simulink model "Praktikum03Grupp09"  (R2023b)
settings: Solver=VariableStepAuto  StartTime=0.0  StopTime=Inf  RelTol=1e-3
model workspace (MAT data in the model file):
  M = 16
  Ts = 5e-08
undefined symbols (not defined in the file): doppler
libraries: commchan3 x6, commrflib2 x6, dspsrcs4 x4, dspxfrm3 x3, commrandsrc3 x2, dspsigops x2, commdigbbndam3 x2, dspstat3 x1, dspmathops x1
settings Model: Creator=suttarar@hu-berlin.de  LastModifiedBy=suttarar@hu-berlin.de

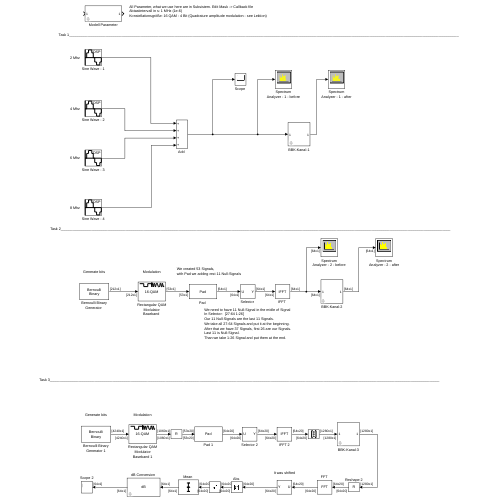
[thumbnail: Simulink's stored preview of the top-level diagram]
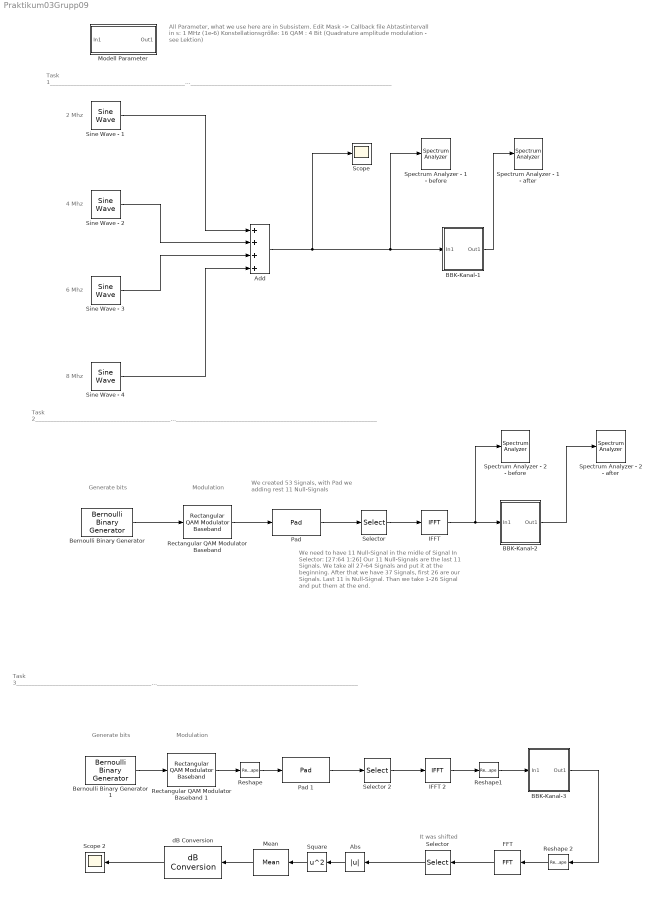
== system Praktikum03Grupp09 ==
  note: It was shifted
  note: Task 1________________________________________________________________________________________________________________________________________________________________________________________________
  note: We need to have 11 Null-Signal in the midle of Signal
      | In Selector:  [27:64 1:26]
      | Our 11 Null-Signals are the last 11 Signals.
      | We take all 27-64 Signals and put it at the beginning.
      | After that we have 37 Signals, first 26 are our Signals.
      | Last 11 is Null-Signal.
      | Than we take 1-26 Signal and put them at the end.
  note: We created 53 Signals,
      | with Pad we adding rest 11 Null-Signals
  note: 2 Mhz
  note: 4 Mhz
  note: 6 Mhz
  note: 8 Mhz
  note: All Parameter, what we use here are in Subsistem. Edit Mask -> Callback file
      | Abtastintervall in s: 1 MHz (1e-6)
      | Konstellationsgröße: 16 QAM : 4 Bit (Quadrature amplitude modulation - see Lektion)
  note: Modulation
  note: Generate bits
  note: Task 2________________________________________________________________________________________________________________________________________________________________________________________________
  note: Generate bits
  note: Task 3________________________________________________________________________________________________________________________________________________________________________________________________
  note: Modulation
  "Abs " : Abs  SaturateOnIntegerOverflow=off
  "Add " : Sum  Inputs=++++
  BBK-Kanal-1 : Subsystem  mask{MaxDoppler=10, PathDelays=[0 100]*1e-9, PathGains=[0 -3], EnableMultipath=1, PathLoss=0, FrequencyOffset=0, PhaseOffset=0, SNR=20}
      mask prompts: MaxDoppler "Dopplerverschiebung"; PathDelays "Pfadverzoergerungen"; PathGains "Pfadverstaerkungen"; EnableMultipath "SwitchBlock"; PathLoss "Pfadverlust"; FrequencyOffset "Frequenzverschiebung"; PhaseOffset "Phasenverschiebung"; SNR "AWG-Rauschen"
  BBK-Kanal-2 : Subsystem  mask{MaxDoppler=10, PathDelays=[0 100]*1e-9, PathGains=[0 -3], EnableMultipath=1, PathLoss=0, FrequencyOffset=0, PhaseOffset=0, SNR=20}
      mask prompts: MaxDoppler "Dopplerverschiebung"; PathDelays "Pfadverzoergerungen"; PathGains "Pfadverstaerkungen"; EnableMultipath "SwitchBlock"; PathLoss "Pfadverlust"; FrequencyOffset "Frequenzverschiebung"; PhaseOffset "Phasenverschiebung"; SNR "AWG-Rauschen"
  BBK-Kanal-3 : Subsystem  mask{MaxDoppler=10, PathDelays=[0 100]*1e-9, PathGains=[0 -3], EnableMultipath=1, PathLoss=0, FrequencyOffset=0, PhaseOffset=0, SNR=20}
      mask prompts: MaxDoppler "Dopplerverschiebung"; PathDelays "Pfadverzoergerungen"; PathGains "Pfadverstaerkungen"; EnableMultipath "SwitchBlock"; PathLoss "Pfadverlust"; FrequencyOffset "Frequenzverschiebung"; PhaseOffset "Phasenverschiebung"; SNR "AWG-Rauschen"
  "Bernoulli Binary Generator " : commrandsrc3/Bernoulli Binary Generator  ProbabilityOfZero=0.5  SeedSource=Auto  Seed=0  SampleTime=Ts*64/(log2(M)*53)  SamplesPerFrame=log2(M)*53  OutputDataType=double  SimulateUsing=Interpreted execution
  Bernoulli Binary Generator 1 : commrandsrc3/Bernoulli Binary Generator  ProbabilityOfZero=0.5  SeedSource=Auto  Seed=0  SampleTime=Ts*64/(log2(M)*53)  SamplesPerFrame=log2(M)*53 * 20  OutputDataType=double  SimulateUsing=Interpreted execution
  "FFT " : dspxfrm3/FFT  FFTImplementation=Auto  CompMethod=Table lookup  TableOpt=NEW  TableOptActive=Speed  BitRevOrder=off  Normalize=off  InheritFFTLength=on  FFTLength=64  WrapInput=on  roundingMode=Floor  overflowMode=off  firstCoeffDataTypeStr=Inherit: Same word length as input  firstCoeffLastDataTypeStr=Inherit: Same word length as input  outputMin=[]  outputMax=[]
  "IFFT " : dspxfrm3/IFFT  FFTImplementation=Auto  CompMethod=Table lookup  TableOpt=NEW  TableOptActive=Speed  BitRevOrder=off  cs_in=off  Normalize=on  InheritFFTLength=on  FFTLength=64  WrapInput=on  mode=Complex  outSamplingMode=Sample based  roundingMode=Floor  overflowMode=off  firstCoeffDataTypeStr=Inherit: Same word length as input  firstCoeffLastDataTypeStr=Inherit: Same word length as input  outputMin=[]  outputMax=[]
  IFFT 2 : dspxfrm3/IFFT  FFTImplementation=Auto  CompMethod=Table lookup  TableOpt=NEW  TableOptActive=Speed  BitRevOrder=off  cs_in=off  Normalize=on  InheritFFTLength=on  FFTLength=64  WrapInput=on  mode=Complex  outSamplingMode=Sample based  roundingMode=Floor  overflowMode=off  firstCoeffDataTypeStr=Inherit: Same word length as input  firstCoeffLastDataTypeStr=Inherit: Same word length as input  outputMin=[]  outputMax=[]
  "Mean " : dspstat3/Mean  run=off  InputProcessing=Columns as channels (frame based)  reset_popup=None  directionMode=Each row  dimension=1  roiEnable=off  roiType=Rectangles  roiPortion=Entire ROI  roiOutput=Individual statistics for each ROI  roiFlag=off  roundingMode=Floor  overflowMode=off  outputDataTypeStr=Inherit: Same as accumulator  outputMin=[]  outputMax=[]  outputLastDataTypeStr=Inherit: Same as accumulator
  Modell Parameter : Subsystem  mask{Ts=1/20e6, M=16}
      mask prompts: Ts "Abtastintervall in s"; M "Konstellationsgröße"
  "Pad " : dspsigops/Pad  padAlong=Columns  dimsToPad=1  valSrc=Specify via dialog  padVal=0  spec=Output size  padNumOutRowsSpecMethod=User-specified  numOutRows=64  padNumOutColsSpecMethod=User-specified  numOutCols=1  isVarDimsMode=off  padBeginning=0  padEnd=0  outSizeMode=User-specified  outSize=1  padSigAt=End  trunc_flag=None  roundingMode=Floor  overflowMode=off  truncOrWrapMode=Truncate  wrap_flag=None
  Pad 1 : dspsigops/Pad  padAlong=Columns  dimsToPad=1  valSrc=Specify via dialog  padVal=0  spec=Output size  padNumOutRowsSpecMethod=User-specified  numOutRows=64  padNumOutColsSpecMethod=User-specified  numOutCols=1  isVarDimsMode=off  padBeginning=0  padEnd=0  outSizeMode=User-specified  outSize=1  padSigAt=End  trunc_flag=None  roundingMode=Floor  overflowMode=off  truncOrWrapMode=Truncate  wrap_flag=None
  "Rectangular QAM Modulator Baseband " : commdigbbndam3/Rectangular QAM Modulator Baseband  M=M  InType=Bit  Enc=Gray  Mapping=[0:15]  PowType=Average Power  MinDist=2  AvgPow=1  PeakPow=1  Ph=0  outDtype=double  outWordLen=16  outUDDataType=sfix(16)  outFracLenMode=Best precision  outFracLen=15  outDataTypeStr=double  outLastDataTypeStr=double
  Rectangular QAM Modulator Baseband 1 : commdigbbndam3/Rectangular QAM Modulator Baseband  M=M  InType=Bit  Enc=Gray  Mapping=[0:15]  PowType=Average Power  MinDist=2  AvgPow=1  PeakPow=1  Ph=0  outDtype=double  outWordLen=16  outUDDataType=sfix(16)  outFracLenMode=Best precision  outFracLen=15  outDataTypeStr=double  outLastDataTypeStr=double
  Reshape : Reshape  OutputDimensionality=Customize  OutputDimensions=[53,20]
  Reshape 2 : Reshape  OutputDimensionality=Customize  OutputDimensions=[64,20]
  Reshape1 : Reshape  OutputDimensionality=Column vector (2-D)  OutputDimensions=[53,20]
  "Scope " : Scope
  Scope 2 : Scope
  Selector : Selector  NumberOfDimensions=2  InputPortWidth=3  IndexOptions=Index vector (dialog),Select all  Indices=[34:64 1:33],1  OutputSizes=1,1
  "Selector " : Selector  NumberOfDimensions=2  InputPortWidth=3  IndexOptions=Index vector (dialog),Select all  Indices=[27:64 1:26],1  OutputSizes=1,1
  Selector 2 : Selector  NumberOfDimensions=2  InputPortWidth=3  IndexOptions=Index vector (dialog),Select all  Indices=[27:64 1:26],1  OutputSizes=1,1
  Sine Wave - 1 : dspsrcs4/Sine Wave  Amplitude=1  Frequency=2e6  Phase=0  SampleMode=Discrete  OutComplex=Complex  CompMethod=Trigonometric fcn  TableSize=Speed  SampleTime=Ts  SamplesPerFrame=1  ResetState=Restart at time zero  OutputFrames=off  dataType=double  wordLen=16  udDataType=sfix(16)  fracBitsMode=Best precision  numFracBits=15  OutDataTypeStr=double  LastOutDataTypeStr=double
  Sine Wave - 2 : dspsrcs4/Sine Wave  Amplitude=1  Frequency=4e6  Phase=0  SampleMode=Discrete  OutComplex=Complex  CompMethod=Trigonometric fcn  TableSize=Speed  SampleTime=Ts  SamplesPerFrame=1  ResetState=Restart at time zero  OutputFrames=off  dataType=double  wordLen=16  udDataType=sfix(16)  fracBitsMode=Best precision  numFracBits=15  OutDataTypeStr=double  LastOutDataTypeStr=double
  Sine Wave - 3 : dspsrcs4/Sine Wave  Amplitude=1  Frequency=6e6  Phase=0  SampleMode=Discrete  OutComplex=Complex  CompMethod=Trigonometric fcn  TableSize=Speed  SampleTime=Ts  SamplesPerFrame=1  ResetState=Restart at time zero  OutputFrames=off  dataType=double  wordLen=16  udDataType=sfix(16)  fracBitsMode=Best precision  numFracBits=15  OutDataTypeStr=double  LastOutDataTypeStr=double
  Sine Wave - 4 : dspsrcs4/Sine Wave  Amplitude=1  Frequency=8e6  Phase=0  SampleMode=Discrete  OutComplex=Complex  CompMethod=Trigonometric fcn  TableSize=Speed  SampleTime=Ts  SamplesPerFrame=1  ResetState=Restart at time zero  OutputFrames=off  dataType=double  wordLen=16  udDataType=sfix(16)  fracBitsMode=Best precision  numFracBits=15  OutDataTypeStr=double  LastOutDataTypeStr=double
  Spectrum Analyzer - 1 - after : SpectrumAnalyzer  WindowPosition=[1074.000000,552.000000,800.000000,500.000000,]  Visible=on  ScopeFrameLocation=window  YLimits=[-32.2048345,40.19991755]
  Spectrum Analyzer - 1 - before : SpectrumAnalyzer  WindowPosition=[154.000000,552.000000,800.000000,500.000000,]  Visible=on  ScopeFrameLocation=window  Span=20000000  StartFrequency=-10000000  StopFrequency=10000000  YLimits=[-49.93409765,38.37141923]
  Spectrum Analyzer - 2 - after : SpectrumAnalyzer  WindowPosition=[1076.000000,31.000000,800.000000,500.000000,]  Visible=on  ScopeFrameLocation=window  Method=Welch  Span=1000  StartFrequency=-500  StopFrequency=500  YLimits=[-25.29856775,-8.25168527]  SelectedToolstripTab=spectrumAnalyzerToolstrip.estimationTab
  Spectrum Analyzer - 2 - before : SpectrumAnalyzer  WindowPosition=[159.000000,31.000000,800.000000,500.000000,]  Visible=on  ScopeFrameLocation=window  Method=Welch  Span=1000  StartFrequency=-500  StopFrequency=500  YLimits=[-58.48285042,-10.3108875]
  Square : Math  Operator=square
  "dB Conversion " : dspmathops/dB Conversion  dBtype=dB  intype=Power  R=1  fuzz=off
      settings: LibrarySourceBlock=commutil2/dB Conversion
  wires:
  Sine Wave - 1/1 -> "Add "/1
  Sine Wave - 2/1 -> "Add "/2
  Sine Wave - 3/1 -> "Add "/3
  Sine Wave - 4/1 -> "Add "/4
  "Add "/1 -> Spectrum Analyzer - 1 - before/1, BBK-Kanal-1/1(In1), "Scope "/1
  BBK-Kanal-1/1(Out1) -> Spectrum Analyzer - 1 - after/1
  "Bernoulli Binary Generator "/1 -> "Rectangular QAM Modulator Baseband "/1
  "Rectangular QAM Modulator Baseband "/1 -> "Pad "/1
  "Selector "/1 -> "IFFT "/1
  "Pad "/1 -> "Selector "/1
  "IFFT "/1 -> Spectrum Analyzer - 2 - before/1, BBK-Kanal-2/1(In1)
  BBK-Kanal-2/1(Out1) -> Spectrum Analyzer - 2 - after/1
  Pad 1/1 -> Selector 2/1
  Selector 2/1 -> IFFT 2/1
  IFFT 2/1 -> Reshape1/1
  Bernoulli Binary Generator 1/1 -> Rectangular QAM Modulator Baseband 1/1
  BBK-Kanal-3/1(Out1) -> Reshape 2/1
  Reshape1/1 -> BBK-Kanal-3/1(In1)
  Rectangular QAM Modulator Baseband 1/1 -> Reshape/1
  Reshape/1 -> Pad 1/1
  Reshape 2/1 -> "FFT "/1
  "FFT "/1 -> Selector/1
  "dB Conversion "/1 -> Scope 2/1
  Square/1 -> "Mean "/1
  "Abs "/1 -> Square/1
  "Mean "/1 -> "dB Conversion "/1
  Selector/1 -> "Abs "/1

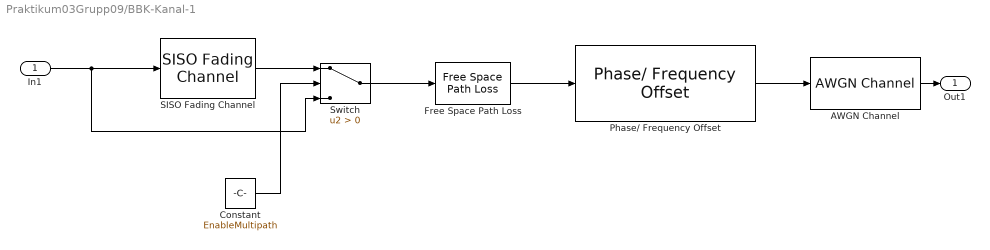
== system Praktikum03Grupp09/BBK-Kanal-1 ==
  In1 : Inport
  AWGN Channel : commchan3/AWGN Channel  LegacyMode=off  NoiseMethod="Signal to noise ratio  (SNR)"  noiseMode="Signal to noise ratio  (SNR)"  EbNo=10  EsNo=10  SNR=SNR  BitsPerSymbol=1  SignalPower=1  SamplesPerSymbol=1  SymbolPeriod=1  VarianceSource=Parameter  Variance=1  RandomStream=Global stream  Seed=67  SimulateUsing=Code generation
  Constant : Constant  Value=EnableMultipath
  Free Space Path Loss : commrflib2/Free Space Path Loss  mode=Decibels  dB=PathLoss  d=0.100  fc=1920
  Phase/ Frequency Offset : commrflib2/Phase// Frequency Offset  phaseOffset=PhaseOffset  freqPort=off  freqOffset=FrequencyOffset
      settings: LibrarySourceBlock=|
      | commrfcorlib/Phase//
      | Frequency
      | Offset
  SISO Fading Channel : commchan3/SISO Fading Channel  InheritSampleRate=on  SampleRate=1  PathDelays=PathDelays  AveragePathGains=PathGains  NormalizePathGains=on  FadingDistribution=Rayleigh  KFactor=3  DirectPathDopplerShift=0  DirectPathInitialPhase=0  MaximumDopplerShift=MaxDoppler  DopplerSpectrum=doppler('Jakes')  RandomStream=mt19937ar with seed  Seed=73  PathGainsOutputPort=off  ChannelFilterDelayOutputPort=off  SimulateUsing=Interpreted execution  Visualization=Off  PathsForDopplerDisplay=1  SamplesToDisplay=25%
  Switch : Switch  Criteria=u2 > Threshold  SaturateOnIntegerOverflow=off  InputSameDT=off
  Out1 : Outport
  wires:
  Phase/ Frequency Offset/1 -> AWGN Channel/1
  Free Space Path Loss/1 -> Phase/ Frequency Offset/1
  AWGN Channel/1 -> Out1/1
  Switch/1 -> Free Space Path Loss/1
  SISO Fading Channel/1 -> Switch/1
  In1/1 -> Switch/3, SISO Fading Channel/1
  Constant/1 -> Switch/2

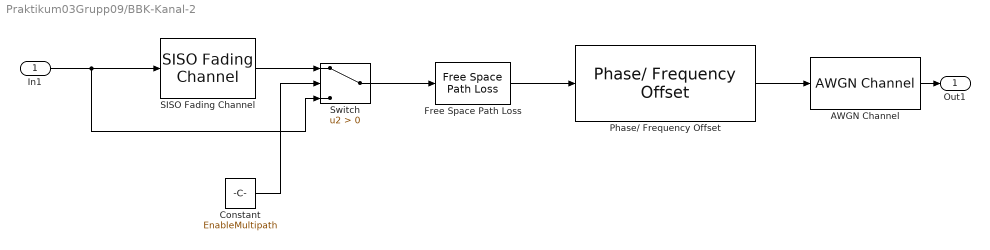
== system Praktikum03Grupp09/BBK-Kanal-2 ==
  In1 : Inport
  AWGN Channel : commchan3/AWGN Channel  LegacyMode=off  NoiseMethod="Signal to noise ratio  (SNR)"  noiseMode="Signal to noise ratio  (SNR)"  EbNo=10  EsNo=10  SNR=SNR  BitsPerSymbol=1  SignalPower=1  SamplesPerSymbol=1  SymbolPeriod=1  VarianceSource=Parameter  Variance=1  RandomStream=Global stream  Seed=67  SimulateUsing=Code generation
  Constant : Constant  Value=EnableMultipath
  Free Space Path Loss : commrflib2/Free Space Path Loss  mode=Decibels  dB=PathLoss  d=0.100  fc=1920
  Phase/ Frequency Offset : commrflib2/Phase// Frequency Offset  phaseOffset=PhaseOffset  freqPort=off  freqOffset=FrequencyOffset
      settings: LibrarySourceBlock=|
      | commrfcorlib/Phase//
      | Frequency
      | Offset
  SISO Fading Channel : commchan3/SISO Fading Channel  InheritSampleRate=on  SampleRate=1  PathDelays=PathDelays  AveragePathGains=PathGains  NormalizePathGains=on  FadingDistribution=Rayleigh  KFactor=3  DirectPathDopplerShift=0  DirectPathInitialPhase=0  MaximumDopplerShift=MaxDoppler  DopplerSpectrum=doppler('Jakes')  RandomStream=mt19937ar with seed  Seed=73  PathGainsOutputPort=off  ChannelFilterDelayOutputPort=off  SimulateUsing=Interpreted execution  Visualization=Off  PathsForDopplerDisplay=1  SamplesToDisplay=25%
  Switch : Switch  Criteria=u2 > Threshold  SaturateOnIntegerOverflow=off  InputSameDT=off
  Out1 : Outport
  wires:
  Phase/ Frequency Offset/1 -> AWGN Channel/1
  Free Space Path Loss/1 -> Phase/ Frequency Offset/1
  AWGN Channel/1 -> Out1/1
  Switch/1 -> Free Space Path Loss/1
  SISO Fading Channel/1 -> Switch/1
  In1/1 -> Switch/3, SISO Fading Channel/1
  Constant/1 -> Switch/2

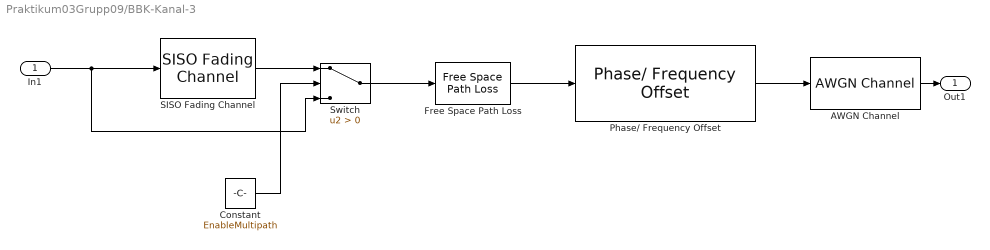
== system Praktikum03Grupp09/BBK-Kanal-3 ==
  In1 : Inport
  AWGN Channel : commchan3/AWGN Channel  LegacyMode=off  NoiseMethod="Signal to noise ratio  (SNR)"  noiseMode="Signal to noise ratio  (SNR)"  EbNo=10  EsNo=10  SNR=SNR  BitsPerSymbol=1  SignalPower=1  SamplesPerSymbol=1  SymbolPeriod=1  VarianceSource=Parameter  Variance=1  RandomStream=Global stream  Seed=67  SimulateUsing=Code generation
  Constant : Constant  Value=EnableMultipath
  Free Space Path Loss : commrflib2/Free Space Path Loss  mode=Decibels  dB=PathLoss  d=0.100  fc=1920
  Phase/ Frequency Offset : commrflib2/Phase// Frequency Offset  phaseOffset=PhaseOffset  freqPort=off  freqOffset=FrequencyOffset
      settings: LibrarySourceBlock=|
      | commrfcorlib/Phase//
      | Frequency
      | Offset
  SISO Fading Channel : commchan3/SISO Fading Channel  InheritSampleRate=on  SampleRate=1  PathDelays=PathDelays  AveragePathGains=PathGains  NormalizePathGains=on  FadingDistribution=Rayleigh  KFactor=3  DirectPathDopplerShift=0  DirectPathInitialPhase=0  MaximumDopplerShift=MaxDoppler  DopplerSpectrum=doppler('Jakes')  RandomStream=mt19937ar with seed  Seed=73  PathGainsOutputPort=off  ChannelFilterDelayOutputPort=off  SimulateUsing=Interpreted execution  Visualization=Off  PathsForDopplerDisplay=1  SamplesToDisplay=25%
  Switch : Switch  Criteria=u2 > Threshold  SaturateOnIntegerOverflow=off  InputSameDT=off
  Out1 : Outport
  wires:
  Phase/ Frequency Offset/1 -> AWGN Channel/1
  Free Space Path Loss/1 -> Phase/ Frequency Offset/1
  AWGN Channel/1 -> Out1/1
  Switch/1 -> Free Space Path Loss/1
  SISO Fading Channel/1 -> Switch/1
  In1/1 -> Switch/3, SISO Fading Channel/1
  Constant/1 -> Switch/2

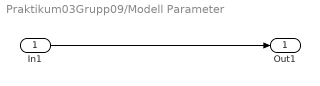
== system Praktikum03Grupp09/Modell Parameter ==
  In1 : Inport
  Out1 : Outport
  wires:
  In1/1 -> Out1/1
